simulink model "MIMODiscreto_2013b"  (Simulink 8.2)
settings: Solver=FixedStepDiscrete  SolverMode=SingleTasking  StartTime=0.0  StopTime=300  FixedStep=0.5  RelTol=1e-3
values from neighbouring files (symbols this model uses):
  Ad = sysZ.A    [MIMOWoodBerry_Discreto.m]    (also in MIMO_Sis.m)
  Bd = sysZ.B    [MIMOWoodBerry_Discreto.m]    (also in MIMO_Sis.m)
  Cd = sysZ.C    [MIMOWoodBerry_Discreto.m]    (also in MIMO_Sis.m)
  Dd = sysZ.D    [MIMOWoodBerry_Discreto.m]    (also in MIMO_Sis.m)
libraries: cstblocks x1
settings Model: Creator=Sergio  LastModifiedBy=Sergio  CovMetricSettings=dwe  CovHtmlReporting=off  covSaveCumulativeToWorkspaceVar=off  CovSaveSingleToWorkspaceVar=off  CovExternalEMLEnable=on
settings DataIOCC: LimitDataPoints=off  SaveFormat=StructureWithTime  SignalLoggingSaveFormat=Dataset
settings OptimizationCC: ExpressionDepthLimit=128
settings DebuggingCC: UnderspecifiedInitializationDetection=Simplified  MergeDetectMultiDrivingBlocksExec=error  SolverPrmCheckMsg=none  FcnCallInpInsideContextMsg=EnableAllAsError  FrameProcessingCompatibilityMsg=error  StateNameClashWarn=none  SFUnexpectedBacktrackingDiag=error  SFNoUnconditionalDefaultTransitionDiag=error
settings HardwareCC: ProdBitPerPointer=64  ProdLargestAtomicFloat=Float  ProdIntDivRoundTo=Zero  ProdEndianess=LittleEndian  ProdHWDeviceType=Specified
settings ModelReferenceCC: PropagateSignalLabelsOutOfModel=on
settings GRTTargetCC: CodeReplacementLibrary=C99 (ISO)  GeneratePreprocessorConditionals=Use local settings  CombineOutputUpdateFcns=on  GRTInterface=off

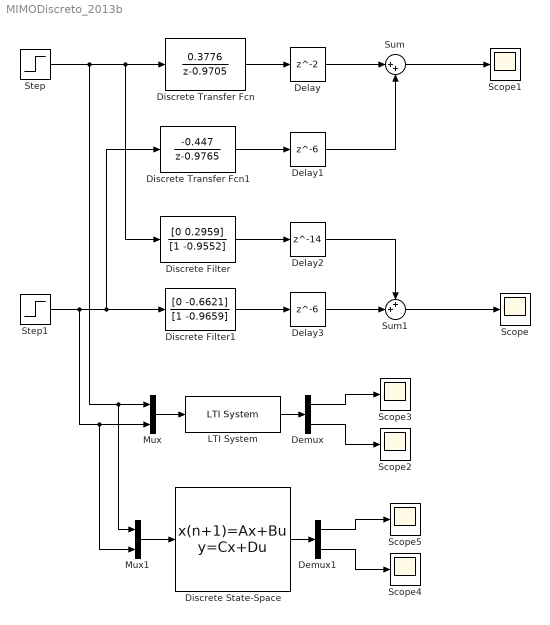
== system MIMODiscreto_2013b ==
  Delay : Delay
  Delay1 : Delay  DelayLength=6  SampleTime=0.5
  Delay2 : Delay  DelayLength=14
  Delay3 : Delay  DelayLength=6
  Demux : Demux  Outputs=2
  Demux1 : Demux  Outputs=2
  Discrete Transfer Fcn : DiscreteTransferFcn  Numerator=[0.3776]  Denominator=[1 -0.9705]  SampleTime=0.5
  Discrete Transfer Fcn1 : DiscreteTransferFcn  Numerator=[-0.447]  Denominator=[1 -0.9765]
  Discrete Filter : DiscreteFilter  Numerator=[0 0.2959]  Denominator=[1 -0.9552]  SampleTime=0.5
  Discrete Filter1 : DiscreteFilter  Numerator=[0 -0.6621]  Denominator=[1 -0.9659]  SampleTime=0.5
  Discrete State-Space : DiscreteStateSpace  A=Ad  B=Bd  C=Cd  D=Dd  SampleTime=0.5
  LTI System : cstblocks/LTI System  sys=Pz  IC=[]
  Mux : Mux  Inputs=2
  Mux1 : Mux  Inputs=2
  Scope{,1..5} (6 alike) : Scope
      Scope settings: TimeRange=auto  MaxDataPoints=5000  SaveToWorkspace=off  SaveName=ScopeData  YMin=-15.21931  YMax=8.85868  SampleTime=-1
      Scope1 settings: TimeRange=auto  MaxDataPoints=5000  SaveToWorkspace=off  YMin=-8.50289  YMax=14.31478  SampleTime=-1
      Scope2 settings: TimeRange=auto  MaxDataPoints=5000  SaveToWorkspace=off  SaveName=ScopeData2  YMin=-15.20582  YMax=8.85237  SampleTime=-1
      Scope3 settings: TimeRange=auto  MaxDataPoints=5000  SaveToWorkspace=off  SaveName=ScopeData3  YMin=-8.36643  YMax=14.29931  SampleTime=-1
      Scope4 settings: TimeRange=auto  MaxDataPoints=5000  SaveToWorkspace=off  SaveName=ScopeData4  YMin=-15.21171  YMax=8.9054  SampleTime=-1
      Scope5 settings: TimeRange=auto  MaxDataPoints=5000  SaveToWorkspace=off  SaveName=ScopeData5  YMin=-8.35425  YMax=14.1895  SampleTime=-1
  Step : Step  Time=5  SampleTime=0.5
  Step1 : Step  Time=50  SampleTime=0.5
  Sum : Sum  Inputs=|++
  Sum1 : Sum  Inputs=++|
  wires:
  Step1/1 -> Mux1/2, Mux/2, Discrete Transfer Fcn1/1, Discrete Filter1/1
  Discrete Filter1/1 -> Delay3/1
  Delay3/1 -> Sum1/2
  Sum1/1 -> Scope/1
  Discrete Filter/1 -> Delay2/1
  Discrete Transfer Fcn1/1 -> Delay1/1
  Discrete Transfer Fcn/1 -> Delay/1
  Delay/1 -> Sum/1
  Sum/1 -> Scope1/1
  Step/1 -> Mux1/1, Mux/1, Discrete Filter/1, Discrete Transfer Fcn/1
  Delay2/1 -> Sum1/1
  Delay1/1 -> Sum/2
  Demux/2 -> Scope2/1
  Demux/1 -> Scope3/1
  LTI System/1 -> Demux/1
  Mux/1 -> LTI System/1
  Discrete State-Space/1 -> Demux1/1
  Demux1/1 -> Scope5/1
  Demux1/2 -> Scope4/1
  Mux1/1 -> Discrete State-Space/1
